simulink model "Pacemaker_group11"  (R2022a)
settings: Solver=FixedStepAuto  StartTime=0.0  StopTime=10.0  FixedStep=1e-3  RelTol=1e-3  EnableMultiTasking=on
undefined symbols (not defined in the file): A0, A1, D0, D1, D10, D11, D12, D13, D2, D3, D4, D5, D6, D7, D8, D9, magnitude, PTA0, PTA1, PTA2, PTB2, PTB23, PTB3, PTB9, PTC16, PTC17, PTC2, PTC3, PTC4, PTD0, PTD1, PTD2, PTD3
libraries: frdmk64flib x20, etargetslib x17, dspstat3 x1, simulink x1
settings Model: ExtModeTrigDuration=5  Creator=12791  LastModifiedBy=39200
settings OptimizationCC: EnhancedBackFolding=on  PassReuseOutputArgsAs=Individual arguments  ZeroExternalMemoryAtStartup=off  ZeroInternalMemoryAtStartup=off  MaxStackSize=64  OptimizeBlockOrder=speed  DifferentSizesBufferReuse=on  OptimizationCustomize=off  EfficientTunableParamExpr=on
settings DebuggingCC: ParameterTunabilityLossMsg=error
settings HardwareCC: ProdBitPerPointer=32  ProdBitPerSizeT=32  ProdBitPerPtrDiffT=32  ProdLargestAtomicInteger=Long  ProdLargestAtomicFloat=Double  ProdWordSize=32  ProdHWDeviceType=ARM Compatible->ARM Cortex
settings SFSimCC: MATLABDynamicMemAlloc=off
settings RTWCC: SystemTargetFile=ert.tlc  HardwareBoard=NXP FRDM-K64F  TLCOptions="-aInlineSetEventsForThisBaseRateFcn=TLC_FALSE -aSuppressMultiTaskScheduler=TLC_FALSE  -aRateBasedStepFcn=0"  TemplateMakefile=ert_default_tmf  Toolchain=GNU Tools for ARM Embedded Processors
settings CodeAppCC: ForceParamTrailComments=on  IgnoreCustomStorageClasses=off  OperatorAnnotations=on  SimulinkDataObjDesc=on  SFDataObjDesc=on  InsertBlockDesc=on
settings ERTTargetCC: ExtModeTransport=4  ExtModeMexFile=sendToCommService

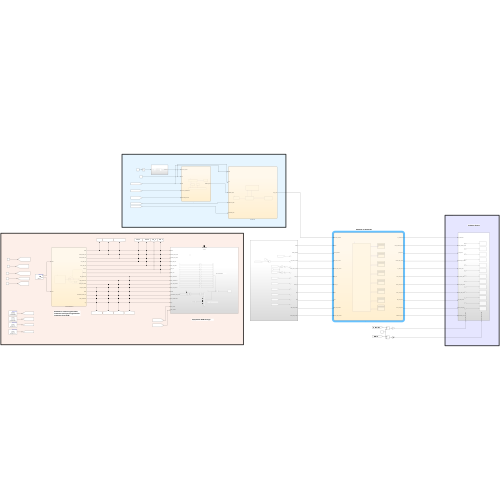
[thumbnail: Simulink's stored preview of the top-level diagram]
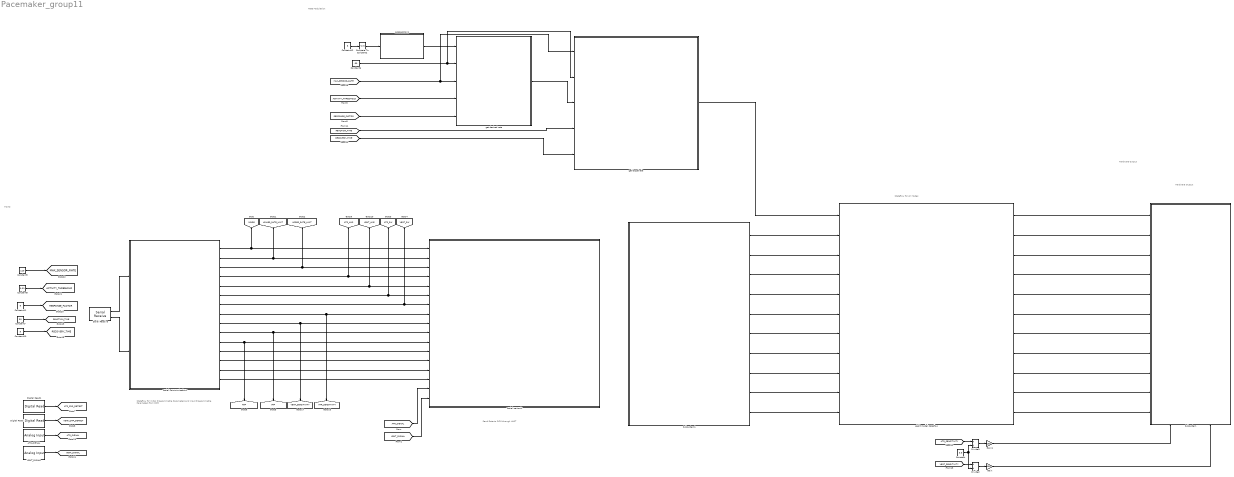
== system Pacemaker_group11 ==
  note: Hardware Output
  note: Rate Modulation
  note: Hardware Output
  note: Inputs
  note: Stateflow for All Modes
  note: Send Data to DCM through UART
  note: Stateflow for Initial Programmable Parameters and Input Programmable Parameters from DCM
  ATR_SIGNAL : frdmk64flib/Analog Input  Whichpin=PTB2 (A0)  SampleTime=-1
  Acceleration1 : Subsystem
  Compare To Constant2 : simulink/Logic and Bit Operations/Compare To Constant  relop=>=  const=5  OutDataTypeStr=boolean
  Constant : Constant  Value=3.3
  Constant10 : Constant  Value=5
  Constant11 : Constant  Value=8
  Constant12 : Constant  Value=5
  Constant6 : Constant  Value=60
  Constant7 : Constant  Value=30
  Constant8 : Constant  Value=0.01
  Constant9 : Constant  Value=120
  Digital Read : frdmk64flib/Digital Read  Whichpin=PTC17 (D1)  SampleTime=-1
  Digital Read1 : frdmk64flib/Digital Read  Whichpin=PTC16 (D0)  SampleTime=-1
  Divide2 : Product  Inputs=*/
  Divide3 : Product  Inputs=*/
  Gain : Gain  Gain=100
  Gain1 : Gain  Gain=100
  Serial Communication1 : Stateflow chart  TreatAsAtomicUnit=on
      settings: PortSchema="{\"entries\":[{\"content\":{\"sides\":[{\"content\":{\"connectorIds\":[\"In1\",\"In2\"]},\"type\":\"ConnectorPlacement.EquallySpacedRectSide\",\"uuid\":\"901574a5-7e09-4852-8827-baac8e876273\"},{\"content\":{\"connectorIds\":[\"Out1\",\"Out2\",\"Out3\",\"Out4\",\"Out12\",\"Out5\",\"Out13\",\"Out14\",\"Out10\",\"Out6\",\"Out11\",\"Out7\",\"Out9\",\"Out8\",\"Out15\"],\"side\":\"RIGHT\"},\"type\":\"ConnectorPlacement.EquallySpacedRectSide\",\"uuid\":\"89d36c37-e833-4dfe-ae0b-2d9eccbce05b\"},{\"content\":{\"connectorIds\":[],\"side\":\"TOP\"},\"type\":\"ConnectorPlacement.EquallySpacedRectSide\",\"uuid\":\"eeb52db1-ccd5-49db-acea-74a4d3271ab8\"}]},\"type\":\"ConnectorPlacement.EquallySpacedConnector\",\"uuid\":\"16ccc146-147c-46a9-b907-deab62e4a6a6\"}],\"packageUris\":[\"http://schema.mathworks.com/mf0/Connector/R2020b\"],\"version\":\"1.0\"}"
  Serial Receive : frdmk64flib/Serial Receive  SCIModule=0  Baudrate=uint32(9600)  Parity=None  StopBits=1  HardwareFlowControl=None  ByteOrder=LittleEndian  DataType=uint8  DataLength=66  BlockingMode=off  OutputStatus=on  SampleTime=-1
  Serial transmit : Subsystem  TreatAsAtomicUnit=on
  Subsystem : Subsystem
      settings: PortSchema="{\"entries\":[{\"content\":{\"sides\":[{\"content\":{\"connectorIds\":[\"In1\",\"In2\",\"In3\",\"In4\",\"In5\",\"In6\",\"In7\",\"In8\",\"In9\",\"In10\",\"In11\"]},\"type\":\"ConnectorPlacement.EquallySpacedRectSide\",\"uuid\":\"cf431d19-a261-4061-b975-82ab8e4554ba\"},{\"content\":{\"connectorIds\":[],\"side\":\"RIGHT\"},\"type\":\"ConnectorPlacement.EquallySpacedRectSide\",\"uuid\":\"d9d96e0a-6018-4f8e-a98f-6eed3a91414e\"},{\"content\":{\"connectorIds\":[],\"side\":\"TOP\"},\"type\":\"ConnectorPlacement.EquallySpacedRectSide\",\"uuid\":\"2358aaff-c3a0-4959-bedb-835f64f1bbed\"},{\"content\":{\"connectorIds\":[\"In12\",\"In13\"],\"side\":\"BOTTOM\"},\"type\":\"ConnectorPlacement.EquallySpacedRectSide\",\"uuid\":\"ece4eb5b-308d-4002-b014-99ad51b61e06\"}]},\"type\":\"ConnectorPlacement.EquallySpacedConnector\",\"uuid\":\"cdbd5127-fb13-4f48-9ecc-e21d40fbaa52\"}],\"packageUris\":[\"http://schema.mathworks.com/mf0/Connector/R2020b\"],\"version\":\"1.0\"}"
  Subsystem1 : Subsystem
  VENT_SIGNAL : frdmk64flib/Analog Input  Whichpin=PTB3 (A1)  SampleTime=-1
  eight model stateflow : Stateflow chart  TreatAsAtomicUnit=on
      settings: PortSchema="{\"entries\":[{\"content\":{\"sides\":[{\"content\":{\"connectorIds\":[\"In6\",\"In7\",\"In2\",\"In4\",\"In1\",\"In8\",\"In9\",\"In11\",\"In10\",\"In5\",\"In3\"]},\"type\":\"ConnectorPlacement.EquallySpacedRectSide\",\"uuid\":\"7bd189cb-d286-447b-b347-38d7b12e59ee\"},{\"content\":{\"connectorIds\":[\"Out1\",\"Out2\",\"Out3\",\"Out4\",\"Out5\",\"Out6\",\"Out7\",\"Out8\",\"Out9\",\"Out10\",\"Out11\"],\"side\":\"RIGHT\"},\"type\":\"ConnectorPlacement.EquallySpacedRectSide\",\"uuid\":\"522f4543-8a7d-441b-9c0c-141bccf5cf26\"},{\"content\":{\"connectorIds\":[],\"side\":\"TOP\"},\"type\":\"ConnectorPlacement.EquallySpacedRectSide\",\"uuid\":\"cf7ae06b-6ef3-498b-825a-38a0a4c90c8a\"}]},\"type\":\"ConnectorPlacement.EquallySpacedConnector\",\"uuid\":\"ae15f7ff-4998-48cc-acd9-270deb6c013f\"}],\"packageUris\":[\"http://schema.mathworks.com/mf0/Connector/R2020b\"],\"version\":\"1.0\"}"
  get desired rate : Stateflow chart  TreatAsAtomicUnit=on
  get target rate : Stateflow chart  TreatAsAtomicUnit=on
      settings: PortSchema="{\"entries\":[{\"content\":{\"sides\":[{\"content\":{\"connectorIds\":[\"In3\",\"In2\",\"In1\",\"In4\",\"In5\"]},\"type\":\"ConnectorPlacement.EquallySpacedRectSide\",\"uuid\":\"b1115713-3752-47d5-be72-104b51cdb1c5\"},{\"content\":{\"connectorIds\":[\"Out1\"],\"side\":\"RIGHT\"},\"type\":\"ConnectorPlacement.EquallySpacedRectSide\",\"uuid\":\"0930a30a-8aa5-4912-ba1f-cc7f148656b0\"},{\"content\":{\"connectorIds\":[],\"side\":\"TOP\"},\"type\":\"ConnectorPlacement.EquallySpacedRectSide\",\"uuid\":\"94dfeeb6-c083-4dc2-b4f5-32fe99d16bb7\"}]},\"type\":\"ConnectorPlacement.EquallySpacedConnector\",\"uuid\":\"5d93a560-4d98-406a-ad12-5273aac4a25c\"}],\"packageUris\":[\"http://schema.mathworks.com/mf0/Connector/R2020b\"],\"version\":\"1.0\"}"
  tag scope: ACTIVITY_THRESHOLD=global, ARP=global, ATR_AMP=global, ATR_CMP_DETECT=global, ATR_PW=global, ATR_SENSITIVITY=global, ATR_SIGNAL=global, LOWER_RATE_LIMIT=global, MAX_SENSOR_RATE=global, MODE=global, REACTION_TIME=global, RECOVERY_TIME=global, RESPONSE_FACTOR=global, UPPER_RATE_LIMIT=global, VENT_AMP=global, VENT_CMP_DETECT=global, VENT_PW=global, VENT_SENSITIVITY=global, VENT_SIGNAL=global, VRP=global
  wires:
  eight model stateflow/1(IS_CHARGING) -> Subsystem/1(IS_CHARGING)
  eight model stateflow/2(PACE_CHARGE_CTRL) -> Subsystem/2(PACE_CHARGE_CTRL)
  eight model stateflow/3(Z_ATR_CTRL) -> Subsystem/3(Z_ATR_CTRL)
  eight model stateflow/4(PACING_REF_PWM) -> Subsystem/4(PACING_REF_PWM)
  eight model stateflow/5(Z_VENT_CTRL) -> Subsystem/5(Z_VENT_CTRL)
  eight model stateflow/6(ATR_PACE_CTRL) -> Subsystem/6(ATR_PACE_CTRL)
  eight model stateflow/7(VENT_PACE_CTRL) -> Subsystem/7(VENT_PACE_CTRL)
  eight model stateflow/9(ATR_GND_CTRL) -> Subsystem/9(ATR_GND_CTRL)
  eight model stateflow/10(VENT_GND_CTRL) -> Subsystem/10(VENT_GND_CTRL)
  eight model stateflow/11(FRONTEND_CTRL) -> Subsystem/11(FRONTEND_CTRL)
  Serial Communication1/1(MODE) -> [MODE], Serial transmit/1(MODE)
  Serial Communication1/2(LOWER_RATE_LIMIT) -> [LOWER_RATE_LIMIT], Serial transmit/2(LOWER_RATE_LIMIT)
  Serial Communication1/3(UPPER_RATE_LIMIT) -> [UPPER_RATE_LIMIT], Serial transmit/3(UPPER_RATE_LIMIT)
  Serial Communication1/5(ATR_PW) -> [ATR_PW], Serial transmit/6(ATR_PW)
  Serial Communication1/13(VENT_PW) -> [VENT_PW], Serial transmit/7(VENT_PW)
  Serial Communication1/14(ATR_SENSITIVITY) -> [ATR_SENSITIVITY], Serial transmit/8(ATR_SENSITIVITY)
  Serial Communication1/10(VENT_SENSITIVITY) -> Serial transmit/9(VENT_SENSITIVITY), [VENT_SENSITIVITY]
  Serial Communication1/7(PVARP) -> Serial transmit/12(PVARP)
  Serial Communication1/9(HYSTERESIS_RATE_LIMIT) -> Serial transmit/13(HYSTERESIS_RATE_LIMIT)
  Serial Communication1/8(RATE_SMOOTHING) -> Serial transmit/14(RATE_SMOOTHING)
  Subsystem1/2(PULSE_PERIOD) -> eight model stateflow/2(PULSE_PERIOD)
  Subsystem1/1(MODE) -> eight model stateflow/7(MODE)
  Subsystem1/4(VENT_DUTY_CYCLE) -> eight model stateflow/1(VENT_DUTY_CYCLE)
  Subsystem1/5(ATR_PW) -> eight model stateflow/8(ATR_PW)
  Subsystem1/6(VENT_PW) -> eight model stateflow/9(VENT_PW)
  Subsystem1/7(ARP) -> eight model stateflow/11(ARP)
  Subsystem1/8(VRP) -> eight model stateflow/10(VRP)
  Subsystem1/3(ATR_DUTY_CYCLE) -> eight model stateflow/4(ATR_DUTY_CYCLE)
  Subsystem1/9(ATR_CMP_DETECT) -> eight model stateflow/5(ATR_CMP_DETECT)
  Subsystem1/10(VENT_CMP_DETECT) -> eight model stateflow/3(VENT_CMP_DETECT)
  Divide2/1 -> Gain/1
  Divide3/1 -> Gain1/1
  Constant/1 -> Divide2/2, Divide3/2
  [VENT_SENSITIVITY] -> Divide2/1
  [ATR_SENSITIVITY] -> Divide3/1
  Gain/1 -> Subsystem/13(VENT_CMP_REF_PWM)
  Gain1/1 -> Subsystem/12(ATR_CMP_REF_PWM)
  Digital Read1/1 -> [ATR_CMP_DETECT]
  Digital Read/1 -> [VENT_CMP_DETECT]
  Serial Communication1/12(VENT_AMP_REG) -> Serial transmit/5(VENT_AMP_REG), [VENT_AMP]
  Serial Communication1/4(ATR_AMP_REG) -> Serial transmit/4(ATR_AMP_REG), [ATR_AMP]
  ATR_SIGNAL/1 -> [ATR_SIGNAL]
  VENT_SIGNAL/1 -> [VENT_SIGNAL]
  Serial Receive/2 -> Serial Communication1/2(status)
  Serial Receive/1 -> Serial Communication1/1(rxdata)
  Serial Communication1/6(VENT_REF_PERIOD) -> Serial transmit/10(VENT_REF_PERIOD), [VRP]
  Serial Communication1/11(ATR_REF_PERIOD) -> [ARP], Serial transmit/11(ATR_REF_PERIOD)
  [VENT_SIGNAL] -> Serial transmit/17(VENT_SIGNAL)
  [ATR_SIGNAL] -> Serial transmit/16(ATR_SIGNAL)
  Serial Communication1/15(Type) -> Serial transmit/15(Type)
  eight model stateflow/8(PACE_GND_CTRL) -> Subsystem/8(PACE_GND_CTRL)
  get target rate/1(Target_rate) -> eight model stateflow/6(MODIFIED_PERIOD)
  [RECOVERY_TIME] -> get target rate/5(RECOVER_TIME)
  [MAX_SENSOR_RATE] -> get desired rate/3(MSR), get target rate/3(MSR)
  get desired rate/1(DESIRED_RATE) -> get target rate/1(DESIRED_RATE)
  Constant7/1 -> [REACTION_TIME]
  [RESPONSE_FACTOR] -> get desired rate/5(RESPONSE_FACTOR)
  Constant11/1 -> [RESPONSE_FACTOR]
  [REACTION_TIME] -> get target rate/4(REACTION_TIME)
  Constant8/1 -> [ACTIVITY_THRESHOLD]
  Constant12/1 -> Compare To Constant2/1
  Compare To Constant2/1 -> Acceleration1/1(In1)
  Constant9/1 -> [MAX_SENSOR_RATE]
  [ACTIVITY_THRESHOLD] -> get desired rate/4(ACTIVITY_THRESHOLD)
  Acceleration1/1(ACTIVITY) -> get desired rate/1(ACTIVITY_LEVEL)
  Constant6/1 -> get desired rate/2(LRL), get target rate/2(LRL)
  Constant10/1 -> [RECOVERY_TIME]

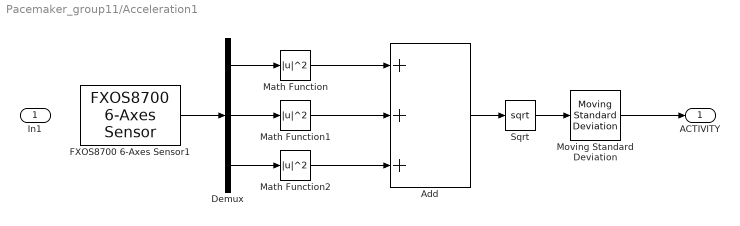
== system Pacemaker_group11/Acceleration1 ==
  In1 : Inport
  Add : Sum  Inputs=+++
  Demux : Demux  Outputs=3
  FXOS8700 6-Axes Sensor1 : frdmk64flib/FXOS8700 6-Axes Sensor  Activesensor=Accelerometer only  ODR=800Hz  HybridODR=400Hz  Accelfullrange=-4g to +4g  SampleTime=-1
  Math Function : Math  Operator=magnitude^2  SignedPower=on  OutDataTypeStr=double
  Math Function1 : Math  Operator=magnitude^2  SignedPower=on  OutDataTypeStr=double
  Math Function2 : Math  Operator=magnitude^2  SignedPower=on  OutDataTypeStr=double
  Moving Standard Deviation : dspstat3/Moving Standard Deviation  Method=Sliding window  ForgettingFactorPort=off  SpecifyWindowLength=on  WindowLength=4  ForgettingFactor=0.9  SimulateUsing=Code generation
      settings: SourceProductBaseCode=DS
  Sqrt : Sqrt
  ACTIVITY : Outport  SourceOfInitialOutputValue=Input signal
  wires:
  Sqrt/1 -> Moving Standard Deviation/1
  Math Function2/1 -> Add/3
  Add/1 -> Sqrt/1
  Math Function1/1 -> Add/2
  Demux/1 -> Math Function/1
  Demux/2 -> Math Function1/1
  Math Function/1 -> Add/1
  FXOS8700 6-Axes Sensor1/1 -> Demux/1
  Demux/3 -> Math Function2/1
  Moving Standard Deviation/1 -> ACTIVITY/1

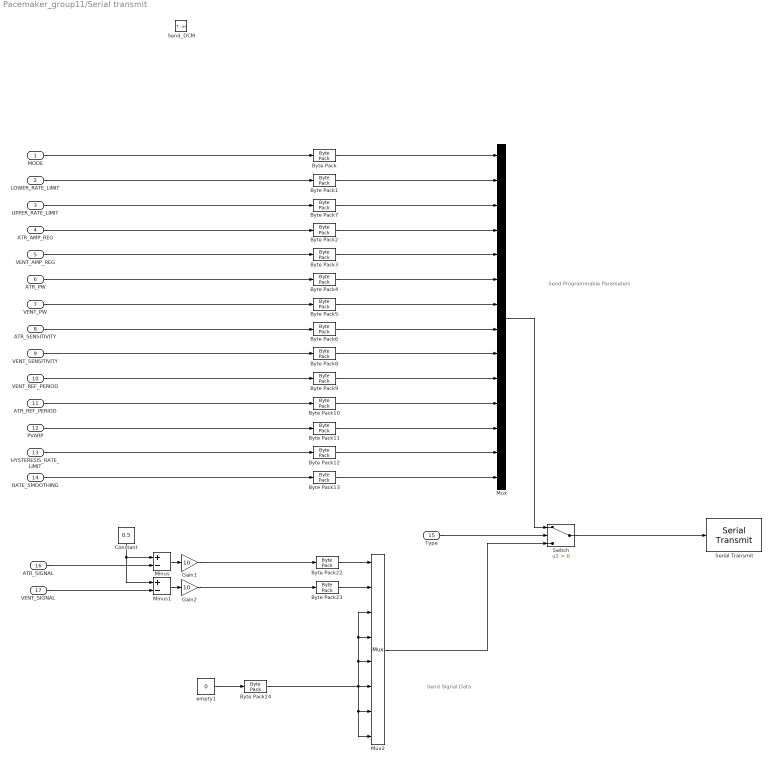
== system Pacemaker_group11/Serial transmit ==
  note: Send Signal Data
  note: Send Programmable Parameters
  MODE : Inport
  LOWER_RATE_LIMIT : Inport  Port=2
  UPPER_RATE_LIMIT : Inport  Port=3
  ATR_AMP_REG : Inport  Port=4
  VENT_AMP_REG : Inport  Port=5
  ATR_PW : Inport  Port=6
  VENT_PW : Inport  Port=7
  ATR_SENSITIVITY : Inport  Port=8
  VENT_SENSITIVITY : Inport  Port=9
  VENT_REF_PERIOD : Inport  Port=10
  ATR_REF_PERIOD : Inport  Port=11
  PVARP : Inport  Port=12
  HYSTERESIS_RATE_LIMIT : Inport  Port=13
  RATE_SMOOTHING : Inport  Port=14
  Type : Inport  Port=15
  ATR_SIGNAL : Inport  Port=16
  VENT_SIGNAL : Inport  Port=17
  Send_DCM : TriggerPort  TriggerType=function-call  IsSimulinkFunction=on  FunctionName=Send_DCM  VariantControl=Variant
  Byte Pack{,1,7,9..13} (8 alike) : etargetslib/Byte Pack  datatypes={'uint16'}  byteAlign=1
  Byte Pack{2..6,8,22..24} (9 alike) : etargetslib/Byte Pack  datatypes={'double'}  byteAlign=1
  Constant : Constant  Value=0.5
  Gain1 : Gain  Gain=10
  Gain2 : Gain  Gain=10
  Minus : Sum  Inputs=+-
  Minus1 : Sum  Inputs=+-
  Mux : Mux  Inputs=14
  Mux2 : Mux  Inputs=8
  Serial Transmit : frdmk64flib/Serial Transmit  SCIModule=0  Baudrate=uint32(9600)  Parity=None  StopBits=1  HardwareFlowControl=None  ByteOrder=LittleEndian  BlockingMode=on  OutputStatus=off
  Switch : Switch  Criteria=u2 > Threshold  SaturateOnIntegerOverflow=off  InputSameDT=off
  empty1 : Constant  Value=0
  wires:
  MODE/1 -> Byte Pack/1
  LOWER_RATE_LIMIT/1 -> Byte Pack1/1
  UPPER_RATE_LIMIT/1 -> Byte Pack7/1
  ATR_AMP_REG/1 -> Byte Pack2/1
  VENT_AMP_REG/1 -> Byte Pack3/1
  ATR_PW/1 -> Byte Pack4/1
  VENT_PW/1 -> Byte Pack5/1
  VENT_SENSITIVITY/1 -> Byte Pack8/1
  ATR_SENSITIVITY/1 -> Byte Pack6/1
  RATE_SMOOTHING/1 -> Byte Pack13/1
  HYSTERESIS_RATE_LIMIT/1 -> Byte Pack12/1
  PVARP/1 -> Byte Pack11/1
  ATR_REF_PERIOD/1 -> Byte Pack10/1
  VENT_REF_PERIOD/1 -> Byte Pack9/1
  Byte Pack1/1 -> Mux/2
  Byte Pack7/1 -> Mux/3
  Byte Pack/1 -> Mux/1
  Byte Pack2/1 -> Mux/4
  Byte Pack3/1 -> Mux/5
  Byte Pack4/1 -> Mux/6
  Byte Pack5/1 -> Mux/7
  Byte Pack6/1 -> Mux/8
  Byte Pack8/1 -> Mux/9
  Byte Pack9/1 -> Mux/10
  Byte Pack10/1 -> Mux/11
  Byte Pack11/1 -> Mux/12
  Byte Pack12/1 -> Mux/13
  Byte Pack13/1 -> Mux/14
  Type/1 -> Switch/2
  Mux/1 -> Switch/1
  Switch/1 -> Serial Transmit/1
  Minus/1 -> Gain1/1
  ATR_SIGNAL/1 -> Minus/2
  Constant/1 -> Minus1/1, Minus/1
  Minus1/1 -> Gain2/1
  VENT_SIGNAL/1 -> Minus1/2
  Gain1/1 -> Byte Pack22/1
  Byte Pack23/1 -> Mux2/2
  Byte Pack24/1 -> Mux2/8, Mux2/7, Mux2/6, Mux2/5, Mux2/3, Mux2/4
  empty1/1 -> Byte Pack24/1
  Mux2/1 -> Switch/3
  Gain2/1 -> Byte Pack23/1
  Byte Pack22/1 -> Mux2/1

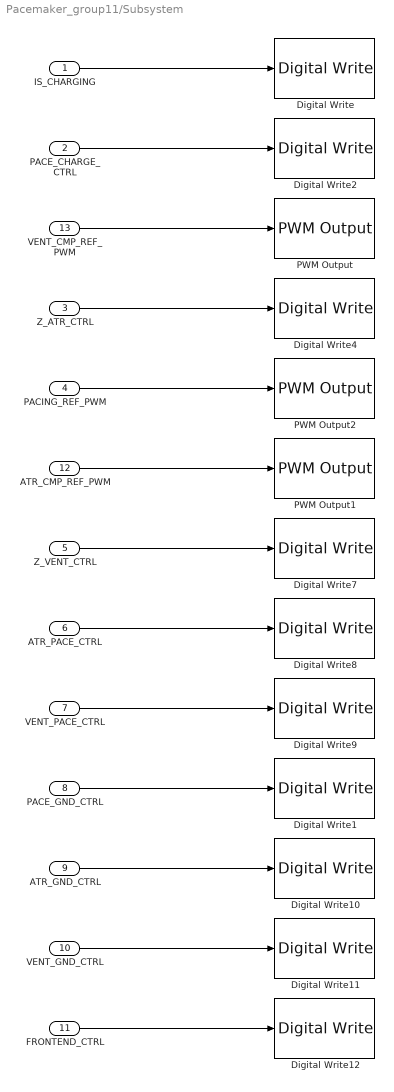
== system Pacemaker_group11/Subsystem ==
  IS_CHARGING : Inport
  PACE_CHARGE_CTRL : Inport  Port=2
  Z_ATR_CTRL : Inport  Port=3
  PACING_REF_PWM : Inport  Port=4
  Z_VENT_CTRL : Inport  Port=5
  ATR_PACE_CTRL : Inport  Port=6
  VENT_PACE_CTRL : Inport  Port=7
  PACE_GND_CTRL : Inport  Port=8
  ATR_GND_CTRL : Inport  Port=9
  VENT_GND_CTRL : Inport  Port=10
  FRONTEND_CTRL : Inport  Port=11
  ATR_CMP_REF_PWM : Inport  Port=12
  VENT_CMP_REF_PWM : Inport  Port=13
  Digital Write : frdmk64flib/Digital Write  Whichpin=RED_LED
  Digital Write1 : frdmk64flib/Digital Write  Whichpin=PTD0 (D10)
  Digital Write10 : frdmk64flib/Digital Write  Whichpin=PTD2 (D11)
  Digital Write11 : frdmk64flib/Digital Write  Whichpin=PTD3 (D12)
  Digital Write12 : frdmk64flib/Digital Write  Whichpin=PTD1 (D13)
  Digital Write2 : frdmk64flib/Digital Write  Whichpin=PTB9 (D2)
  Digital Write4 : frdmk64flib/Digital Write  Whichpin=PTB23 (D4)
  Digital Write7 : frdmk64flib/Digital Write  Whichpin=PTC3 (D7)
  Digital Write8 : frdmk64flib/Digital Write  Whichpin=PTA0 (D8)
  Digital Write9 : frdmk64flib/Digital Write  Whichpin=PTC4 (D9)
  PWM Output : frdmk64flib/PWM Output  Whichpin=PTA1 (D3)  InitialFrequency=2000  InitialDutyCycle=0
  PWM Output1 : frdmk64flib/PWM Output  Whichpin=PTC2 (D6)  InitialFrequency=2000  InitialDutyCycle=0
  PWM Output2 : frdmk64flib/PWM Output  Whichpin=PTA2 (D5)  InitialFrequency=2000  InitialDutyCycle=0
  wires:
  PACE_GND_CTRL/1 -> Digital Write1/1
  Z_ATR_CTRL/1 -> Digital Write4/1
  IS_CHARGING/1 -> Digital Write/1
  PACE_CHARGE_CTRL/1 -> Digital Write2/1
  ATR_PACE_CTRL/1 -> Digital Write8/1
  Z_VENT_CTRL/1 -> Digital Write7/1
  VENT_PACE_CTRL/1 -> Digital Write9/1
  ATR_GND_CTRL/1 -> Digital Write10/1
  PACING_REF_PWM/1 -> PWM Output2/1
  VENT_CMP_REF_PWM/1 -> PWM Output/1
  ATR_CMP_REF_PWM/1 -> PWM Output1/1
  FRONTEND_CTRL/1 -> Digital Write12/1
  VENT_GND_CTRL/1 -> Digital Write11/1

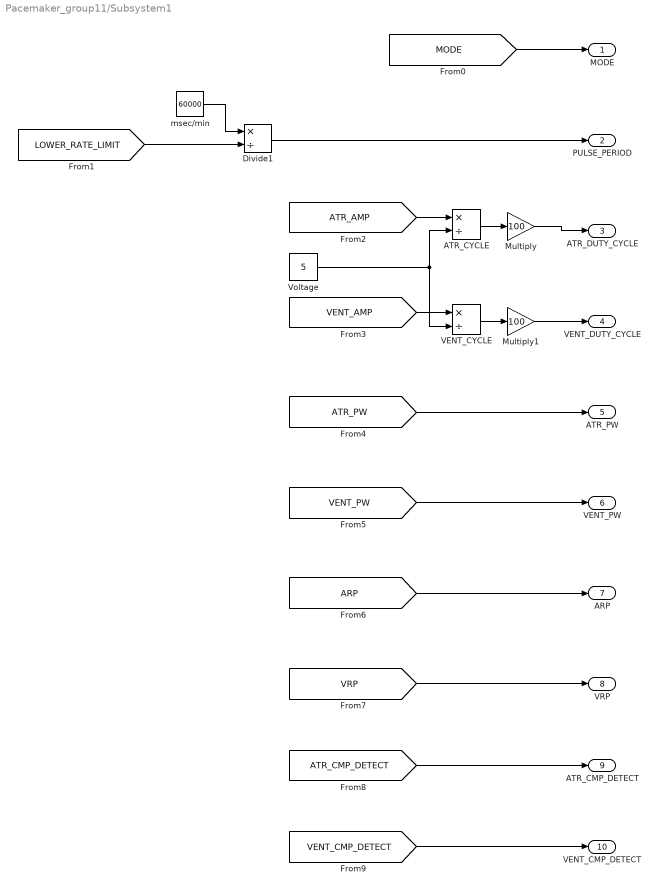
== system Pacemaker_group11/Subsystem1 ==
  ATR_CYCLE : Product  Inputs=*/
  Divide1 : Product  Inputs=*/
  Multiply : Gain  Gain=100
  Multiply1 : Gain  Gain=100
  VENT_CYCLE : Product  Inputs=*/
  Voltage : Constant  Value=5
  msec/min : Constant  Value=60000  OutDataTypeStr=double  LockScale=on
  MODE : Outport
  PULSE_PERIOD : Outport  Port=2
  ATR_DUTY_CYCLE : Outport  Port=3
  VENT_DUTY_CYCLE : Outport  Port=4
  ATR_PW : Outport  Port=5
  VENT_PW : Outport  Port=6
  ARP : Outport  Port=7
  VRP : Outport  Port=8
  ATR_CMP_DETECT : Outport  Port=9
  VENT_CMP_DETECT : Outport  Port=10
  wires:
  msec/min/1 -> Divide1/1
  [LOWER_RATE_LIMIT] -> Divide1/2
  Divide1/1 -> PULSE_PERIOD/1
  Voltage/1 -> VENT_CYCLE/2, ATR_CYCLE/2
  ATR_CYCLE/1 -> Multiply/1
  VENT_CYCLE/1 -> Multiply1/1
  [MODE] -> MODE/1
  Multiply1/1 -> VENT_DUTY_CYCLE/1
  Multiply/1 -> ATR_DUTY_CYCLE/1
  [ATR_AMP] -> ATR_CYCLE/1
  [VENT_AMP] -> VENT_CYCLE/1
  [ATR_PW] -> ATR_PW/1
  [VENT_PW] -> VENT_PW/1
  [ARP] -> ARP/1
  [VRP] -> VRP/1
  [ATR_CMP_DETECT] -> ATR_CMP_DETECT/1
  [VENT_CMP_DETECT] -> VENT_CMP_DETECT/1

== stateflow chart Pacemaker_group11/Serial Communication1 ==
  state SettingParameters
    entry:
    MODE = typecast(rxdata(3:4), 'uint16');
    LOWER_RATE_LIMIT = typecast(rxdata(5:6), 'uint16'); % ppm
    UPPER_RATE_LIMIT = typecast(rxdata(7:8), 'uint16'); % ppm
    ATR_AMP_REG =  typecast(rxdata(9:16), 'double'); % V
    VENT_AMP_REG = typecast(rxdata(17:24), 'double'); % V
    ATR_PW = typecast(rxdata(25:32), 'double'); % ms
    VENT_PW = typecast(rxdata(33:40), 'double'); % ms
    ATR_SENSITIVITY = typecast(rxdata(41:48), 'double'); % mV
    VENT_SENSITIVITY = typecast(rxdata(49:56), 'double'); % mV
    ATR_REF_PERIOD = typecast(rxdata(57:58), 'uint16'); % ms
    VENT_REF_PERIOD = typecast(rxdata(59:60), 'uint16'); % ms
    PVARP = typecast(rxdata(61:62), 'uint16'); % ms
    HYSTERESIS_RATE_LIMIT = typecast(rxdata(63:64), 'uint16'); % ms
    RATE_SMOOTHING = typecast(rxdata(65:66), 'uint16'); % percentage
  state Init
    entry:
    MODE = 0;
    LOWER_RATE_LIMIT = 60;
    UPPER_RATE_LIMIT = 120;
    %MAX_SENSOR_RATE = typecast(rxdata(7:8), 'uint16'); % ppm
    %FIXED_AV_DELAY = typecast(rxdata(9:10), 'uint16'); % ms
    %DYNAMIC_AV_DELAY = rxdata(11); % boolean
    %MIN_DYNAMIC_AV_DELAY =  typecast(rxdata(12:13), 'uint16'); % ms
    %SENSED_AV_DELAY_OFFSET = typecast(rxdata(14:15), 'uint16'); % ms
    ATR_AMP_REG =  3.5; % V
    VENT_AMP_REG = 3.5; % V
    %ATR_AMP_UNREG = typecast(rxdata(9:16), 'double'); % V
    %VENT_AMP_UNREG = typecast(rxdata(9:16), 'double'); % V
    ATR_PW = 0.4; % ms
    VENT_PW = 0.4; % ms
    ATR_SENSITIVITY = 0.75; % mV
    VENT_SENSITIVITY = 2.5; % mV
    ATR_REF_PERIOD = 250; % ms
    VENT_REF_PERIOD = 320; % ms
    PVARP = 250; % ms
    %PVARP_EXTENSION = typecast(rxdata(14:15), 'uint16'); % ms
    HYSTERESIS_RATE_LIMIT = 0; % ms
    RATE_SMOOTHING = 0; % percentage
  state STANDBY
    %Waiting for COM
  state ECHO_PARAM1
    entry:
    Type = 0
    Send_DCM();
  state ECHO_PARAM
    entry:
    Type = 1
    Send_DCM();
  (default) -> Init
  SettingParameters -> STANDBY
  (junction 96) -> STANDBY [order 2]
  (junction 94) -> SettingParameters [order 3] : [rxdata(2) == hex2dec('55')]
  STANDBY -> (junction 96) : [status == 0]
  (junction 96) -> (junction 94) [order 1] : [rxdata(1) == hex2dec('16')]
  Init -> STANDBY
  (junction 94) -> ECHO_PARAM [order 1] : [rxdata(2) == hex2dec('22')]
  (junction 94) -> ECHO_PARAM1 [order 2] : [rxdata(2) == hex2dec('33')]
  ECHO_PARAM -> STANDBY
  ECHO_PARAM1 -> STANDBY
  data: MODE output uint16; LOWER_RATE_LIMIT output uint16; UPPER_RATE_LIMIT output uint16; ATR_AMP_REG output double; ATR_PW output double; rxdata input uint8; status input uint8; VENT_REF_PERIOD output uint16; PVARP output uint16; RATE_SMOOTHING output uint16; HYSTERESIS_RATE_LIMIT output uint16; VENT_SENSITIVITY output double; ATR_REF_PERIOD output uint16; VENT_AMP_REG output double; VENT_PW output double; ATR_SENSITIVITY output; Type output

== stateflow chart Pacemaker_group11/eight model stateflow ==
  state Start
  state AOO [group]
    state Charging_C22
      entry:
      %Charging C22 and discharging C21
      PACING_REF_PWM = ATR_DUTY_CYCLE
      PACE_CHARGE_CTRL = true
      PACE_GND_CTRL = true
      ATR_PACE_CTRL = false
      Z_ATR_CTRL = false
      Z_VENT_CTRL = false
      VENT_PACE_CTRL = false
      VENT_GND_CTRL = false
      ATR_GND_CTRL = true
      % For LED testing
      IS_CHARGING = true
    state Pacing
      entry:
      PACE_CHARGE_CTRL = false
      PACE_GND_CTRL = true
      VENT_PACE_CTRL = false
      VENT_GND_CTRL = false
      Z_ATR_CTRL = false
      Z_VENT_CTRL = false
      ATR_GND_CTRL = false
      ATR_PACE_CTRL = true
      % For LED testing
      IS_CHARGING = false
    AOO.Charging_C22 -> AOO.Pacing [order 1] : [after(PULSE_PERIOD-ATR_PW,msec)]
    AOO.Pacing -> AOO.Charging_C22 : [after(ATR_PW,msec)]
  state VOO [group]
    state Charging_C22
      entry:
      %Charging C22 and discharging C21
      PACING_REF_PWM = VENT_DUTY_CYCLE
      PACE_CHARGE_CTRL = true
      PACE_GND_CTRL = true
      VENT_PACE_CTRL = false
      Z_ATR_CTRL = false
      Z_VENT_CTRL = false
      ATR_PACE_CTRL = false
      ATR_GND_CTRL = false
      VENT_GND_CTRL = true
      % For LED testing
      IS_CHARGING = true
    state Pacing
      entry:
      PACE_CHARGE_CTRL = false
      PACE_GND_CTRL = true
      ATR_PACE_CTRL = false
      ATR_GND_CTRL = false
      Z_ATR_CTRL = false
      Z_VENT_CTRL = false
      VENT_GND_CTRL = false
      VENT_PACE_CTRL = true
      % For LED testing
      IS_CHARGING = false
    VOO.Charging_C22 -> VOO.Pacing [order 1] : [after(PULSE_PERIOD-VENT_PW,msec)]
    VOO.Pacing -> VOO.Charging_C22 : [after(VENT_PW,msec)]
  state AAI [group]
    state Charging_C22
      entry:
      %Charging C22 and discharging C21
      PACING_REF_PWM = ATR_DUTY_CYCLE
      PACE_CHARGE_CTRL = true
      PACE_GND_CTRL = true
      ATR_PACE_CTRL = false
      Z_ATR_CTRL = false
      Z_VENT_CTRL = false
      VENT_PACE_CTRL = false
      VENT_GND_CTRL = false
      ATR_GND_CTRL = true
      % For LED testing
      IS_CHARGING = true
      FRONTEND_CTRL = true
    state Proxy
      entry:
      %Charging C22 and discharging C21
      PACING_REF_PWM = ATR_DUTY_CYCLE
      PACE_CHARGE_CTRL = true
      PACE_GND_CTRL = true
      ATR_PACE_CTRL = false
      Z_ATR_CTRL = false
      Z_VENT_CTRL = false
      VENT_PACE_CTRL = false
      VENT_GND_CTRL = false
      ATR_GND_CTRL = true
      % For LED testing
      IS_CHARGING = true
    state Pacing
      entry:
      PACE_CHARGE_CTRL = false
      PACE_GND_CTRL = true
      VENT_PACE_CTRL = false
      VENT_GND_CTRL = false
      Z_ATR_CTRL = false
      Z_VENT_CTRL = false
      ATR_GND_CTRL = false
      ATR_PACE_CTRL = true
      % For LED testing
      IS_CHARGING = false
    AAI.Charging_C22 -> AAI.Proxy [order 1] : [ATR_CMP_DETECT ==  true]{DELAY = ARP}
    AAI.Proxy -> AAI.Charging_C22 : [after(DELAY,msec)]
    AAI.Charging_C22 -> AAI.Pacing [order 2] : [after(PULSE_PERIOD-ARP,msec)]
    AAI.Pacing -> AAI.Proxy : [after(ATR_PW,msec)]{DELAY = ARP - ATR_PW }
  state VVI [group]
    state Charging_C22
      entry:
      %Charging C22 and discharging C21
      PACING_REF_PWM = VENT_DUTY_CYCLE
      PACE_CHARGE_CTRL = true
      PACE_GND_CTRL = true
      VENT_PACE_CTRL = false
      Z_ATR_CTRL = false
      Z_VENT_CTRL = false
      ATR_PACE_CTRL = false
      ATR_GND_CTRL = false
      VENT_GND_CTRL = true
      % For LED testing
      IS_CHARGING = true
      FRONTEND_CTRL = true
    state Proxy
      entry:
      %Charging C22 and discharging C21
      PACING_REF_PWM = VENT_DUTY_CYCLE
      PACE_CHARGE_CTRL = true
      PACE_GND_CTRL = true
      VENT_PACE_CTRL = false
      Z_ATR_CTRL = false
      Z_VENT_CTRL = false
      ATR_PACE_CTRL = false
      ATR_GND_CTRL = false
      VENT_GND_CTRL = true
      % For LED testing
      IS_CHARGING = true
    state Pacing
      entry:
      PACE_CHARGE_CTRL = false
      PACE_GND_CTRL = true
      ATR_PACE_CTRL = false
      ATR_GND_CTRL = false
      Z_ATR_CTRL = false
      Z_VENT_CTRL = false
      VENT_GND_CTRL = false
      VENT_PACE_CTRL = true
      % For LED testing
      IS_CHARGING = false
    VVI.Charging_C22 -> VVI.Proxy [order 1] : [VENT_CMP_DETECT ==  true]{DELAY = VRP}
    VVI.Proxy -> VVI.Charging_C22 : [after(DELAY,msec)]
    VVI.Charging_C22 -> VVI.Pacing [order 2] : [after(PULSE_PERIOD-VRP,msec)]
    VVI.Pacing -> VVI.Proxy : [after(VENT_PW,msec)]{DELAY = VRP - VENT_PW }
  state AOOR [group]
    state Charging_C22
      entry:
      PACING_REF_PWM = ATR_DUTY_CYCLE
      PACE_CHARGE_CTRL = true
      PACE_GND_CTRL = true
      ATR_PACE_CTRL = false
      Z_ATR_CTRL = false
      Z_VENT_CTRL = false
      VENT_PACE_CTRL = false
      VENT_GND_CTRL = false
      ATR_GND_CTRL = true
      % For LED testing
      IS_CHARGING = true
    state Pacing
      entry:
      PACE_CHARGE_CTRL = false
      PACE_GND_CTRL = true
      VENT_PACE_CTRL = false
      VENT_GND_CTRL = false
      Z_ATR_CTRL = false
      Z_VENT_CTRL = false
      ATR_GND_CTRL = false
      ATR_PACE_CTRL = true
      % For LED testing
      IS_CHARGING = false
    AOOR.Charging_C22 -> AOOR.Pacing [order 1] : [after(MODIFIED_PERIOD-ATR_PW,msec)]
    AOOR.Pacing -> AOOR.Charging_C22 : [after(ATR_PW,msec)]
  state VOOR [group]
    state Charging_C22
      entry:
      PACING_REF_PWM = VENT_DUTY_CYCLE
      PACE_CHARGE_CTRL = true
      PACE_GND_CTRL = true
      VENT_PACE_CTRL = false
      Z_ATR_CTRL = false
      Z_VENT_CTRL = false
      ATR_PACE_CTRL = false
      ATR_GND_CTRL = false
      VENT_GND_CTRL = true
      % For LED testing
      IS_CHARGING = true
    state Pacing
      entry:
      PACE_CHARGE_CTRL = false
      PACE_GND_CTRL = true
      ATR_PACE_CTRL = false
      ATR_GND_CTRL = false
      Z_ATR_CTRL = false
      Z_VENT_CTRL = false
      VENT_GND_CTRL = false
      VENT_PACE_CTRL = true
      % For LED testing
      IS_CHARGING = false
    VOOR.Charging_C22 -> VOOR.Pacing [order 1] : [after(MODIFIED_PERIOD-VENT_PW,msec)]
    VOOR.Pacing -> VOOR.Charging_C22 : [after(VENT_PW,msec)]
  state AAIR [group]
    state Charging_C22
      entry:
      PACING_REF_PWM = ATR_DUTY_CYCLE
      PACE_CHARGE_CTRL = true
      PACE_GND_CTRL = true
      ATR_PACE_CTRL = false
      Z_ATR_CTRL = false
      Z_VENT_CTRL = false
      VENT_PACE_CTRL = false
      VENT_GND_CTRL = false
      ATR_GND_CTRL = true
      % For LED testing
      IS_CHARGING = true
      FRONTEND_CTRL = true
    state Proxy
      entry:
      PACING_REF_PWM = ATR_DUTY_CYCLE
      PACE_CHARGE_CTRL = true
      PACE_GND_CTRL = true
      ATR_PACE_CTRL = false
      Z_ATR_CTRL = false
      Z_VENT_CTRL = false
      VENT_PACE_CTRL = false
      VENT_GND_CTRL = false
      ATR_GND_CTRL = true
      % For LED testing
      IS_CHARGING = true
    state Pacing
      entry:
      PACE_CHARGE_CTRL = false
      PACE_GND_CTRL = true
      VENT_PACE_CTRL = false
      VENT_GND_CTRL = false
      Z_ATR_CTRL = false
      Z_VENT_CTRL = false
      ATR_GND_CTRL = false
      ATR_PACE_CTRL = true
      % For LED testing
      IS_CHARGING = false
    AAIR.Charging_C22 -> AAIR.Proxy [order 1] : [ATR_CMP_DETECT ==  true]{DELAY = ARP}
    AAIR.Proxy -> AAIR.Charging_C22 : [after(DELAY,msec)]
    AAIR.Charging_C22 -> AAIR.Pacing [order 2] : [after(MODIFIED_PERIOD-ARP,msec)]
    AAIR.Pacing -> AAIR.Proxy : [after(ATR_PW,msec)]{DELAY = ARP - ATR_PW }
  state VVIR [group]
    state Charging_C22
      entry:
      PACING_REF_PWM = VENT_DUTY_CYCLE
      PACE_CHARGE_CTRL = true
      PACE_GND_CTRL = true
      VENT_PACE_CTRL = false
      Z_ATR_CTRL = false
      Z_VENT_CTRL = false
      ATR_PACE_CTRL = false
      ATR_GND_CTRL = false
      VENT_GND_CTRL = true
      % For LED testing
      IS_CHARGING = true
      FRONTEND_CTRL = true
    state Proxy
      entry:
      PACING_REF_PWM = VENT_DUTY_CYCLE
      PACE_CHARGE_CTRL = true
      PACE_GND_CTRL = true
      VENT_PACE_CTRL = false
      Z_ATR_CTRL = false
      Z_VENT_CTRL = false
      ATR_PACE_CTRL = false
      ATR_GND_CTRL = false
      VENT_GND_CTRL = true
      % For LED testing
      IS_CHARGING = true
    state Pacing
      entry:
      PACE_CHARGE_CTRL = false
      PACE_GND_CTRL = true
      ATR_PACE_CTRL = false
      ATR_GND_CTRL = false
      Z_ATR_CTRL = false
      Z_VENT_CTRL = false
      VENT_GND_CTRL = false
      VENT_PACE_CTRL = true
      % For LED testing
      IS_CHARGING = false
    VVIR.Charging_C22 -> VVIR.Proxy [order 1] : [VENT_CMP_DETECT ==  true]{DELAY = VRP}
    VVIR.Proxy -> VVIR.Charging_C22 : [after(DELAY,msec)]
    VVIR.Charging_C22 -> VVIR.Pacing [order 2] : [after(MODIFIED_PERIOD-VRP,msec)]
    VVIR.Pacing -> VVIR.Proxy : [after(VENT_PW,msec)]{DELAY = VRP - VENT_PW }
  VOOR.Charging_C22 -> Start [order 2] : [MODE ~= 6]
  VVIR.Charging_C22 -> Start [order 3] : [MODE ~= 8]
  AAIR.Charging_C22 -> Start [order 3] : [MODE ~= 7]
  Start -> AOO.Charging_C22 [order 2] : [MODE == 1]
  Start -> VOO.Charging_C22 [order 1] : [MODE == 2]
  AOOR.Charging_C22 -> Start [order 2] : [MODE ~= 5]
  Start -> VVI.Charging_C22 [order 7] : [MODE == 4]
  Start -> AOOR.Charging_C22 [order 4] : [MODE == 5]
  (default) -> Start
  Start -> VOOR.Charging_C22 [order 8] : [MODE == 6]
  VVI.Charging_C22 -> Start [order 3] : [MODE ~= 4]
  Start -> AAI.Charging_C22 [order 3] : [MODE == 3]
  AAI.Charging_C22 -> Start [order 3] : [MODE ~= 3]
  AOO.Charging_C22 -> Start [order 2] : [MODE ~= 1]
  VOO.Charging_C22 -> Start [order 2] : [MODE ~= 2]
  Start -> AAIR.Charging_C22 [order 5] : [MODE == 7]
  Start -> VVIR.Charging_C22 [order 6] : [MODE == 8]
  data: IS_CHARGING output; PACE_CHARGE_CTRL output; Z_ATR_CTRL output; PACING_REF_PWM output; Z_VENT_CTRL output; ATR_PACE_CTRL output; VENT_PACE_CTRL output; PACE_GND_CTRL output; ATR_GND_CTRL output; VENT_GND_CTRL output; FRONTEND_CTRL output =true; VENT_DUTY_CYCLE input; PULSE_PERIOD input; VENT_CMP_DETECT input; DELAY local; ATR_DUTY_CYCLE input; ATR_CMP_DETECT input; MODIFIED_PERIOD input; MODE input; ATR_PW input; VENT_PW input; VRP input; ARP input

== stateflow chart Pacemaker_group11/get desired rate ==
  state check
    %check if the actvity level below the threshold
  state Desires_output_1
    entry:
    DESIRED_RATE=LRL;
  state Desires_output_3
    entry:
    DESIRED_RATE = Local_rate;
  state Desires_output_2
    entry:
    DESIRED_RATE = MSR;
  state Increase_Linear
    entry:
    Local_rate = LRL + RESPONSE_FACTOR*(ACTIVITY_LEVEL-ACTIVITY_THRESHOLD);
  (default) -> check
  check -> Desires_output_1 [order 1] : [ACTIVITY_LEVEL<=ACTIVITY_THRESHOLD]
  Desires_output_1 -> check : after(100,msec)
  check -> Increase_Linear [order 2] : [ACTIVITY_LEVEL>ACTIVITY_THRESHOLD]
  Desires_output_3 -> check : after(100,msec)
  Desires_output_2 -> check : after(100,msec)
  Increase_Linear -> Desires_output_2 [order 1] : [Local_rate >=MSR]
  Increase_Linear -> Desires_output_3 [order 2] : [Local_rate<MSR]
  data: ACTIVITY_LEVEL input; LRL input; MSR input; ACTIVITY_THRESHOLD input; RESPONSE_FACTOR input; DESIRED_RATE output; Local_rate local

== stateflow chart Pacemaker_group11/get target rate ==
  state increase_state
    entry:
    %use linear:
    if(Target_rate<MSR && Target_rate<DESIRED_RATE)
    Target_rate=Target_rate+step_up;
    elseif(Target_rate == DESIRED_RATE)
    Target_rate = DESIRED_RATE;
    elseif(Target_rate>MSR)
    Target_rate = MSR
    end
  state step_state
    entry:
    step_up = (MSR-LRL)/REACTION_TIME;
    step_down = (MSR-LRL)/RECOVER_TIME;
  state decrease_state
    entry:
    if(Target_rate<MSR)
    Target_rate = Target_rate - step_down;
    elseif(Target_rate <= LRL)
    Target_rate = LRL;
    end
  state start_state
    %set target rate to at least LRL
    Target_rate = LRL;
  step_state -> increase_state [order 2] : after(100,msec)[Target_rate<=DESIRED_RATE]
  increase_state -> step_state : after(100,msec)
  (default) -> start_state
  step_state -> decrease_state [order 1] : after(100,msec)[Target_rate>DESIRED_RATE]
  decrease_state -> step_state : after(100,msec)
  start_state -> step_state : [Target_rate>=LRL]
  data: DESIRED_RATE input; Target_rate output; LRL input; MSR input; REACTION_TIME input; RECOVER_TIME input; step_down local; step_up local
